simulink model "soc_estimation"  (R2024a)
settings: Solver=ode4  StartTime=0.0  StopTime=25000  FixedStep=0.001  MinStep=1e-3  RelTol=1e-3
values from neighbouring files (symbols this model uses):
  C1 = 1.6e-6    (= 1.6e-06)    [model_parameters.m]
  g = 9.8    [model_parameters.m]
  m = 860    [model_parameters.m]
  r = 0.33    [model_parameters.m]
  rho = 1.2    [model_parameters.m]
  S = 2.75    [model_parameters.m]
undefined symbols (not defined in the file or in its folder): C0, Cx
libraries: drivecyclelib x1
settings Model: Creator=marco  LastModifiedBy=QUDUS
settings SolverCC: AlgebraicLoopSolver=TrustRegion
settings DataIOCC: ReturnWorkspaceOutputs=off
settings DebuggingCC: UnconnectedInputMsg=warning  UnconnectedOutputMsg=warning  UnconnectedLineMsg=warning  UnderSpecifiedDimensionMsg=warning  ArithmeticOperatorsInVariantConditions=warning
settings ModelReferenceCC: EnableRefExpFcnMdlSchedulingChecks=on
settings SFSimCC: CustomCodeUndefinedFunction=UseInterfaceOnly
settings RTWCC: GPUComputeCapability=3.5

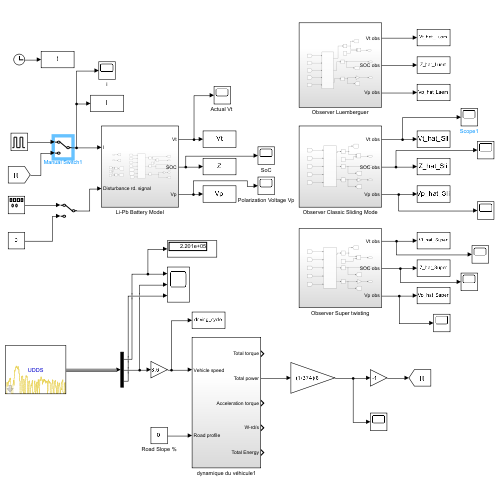
[thumbnail: Simulink's stored preview of the top-level diagram]
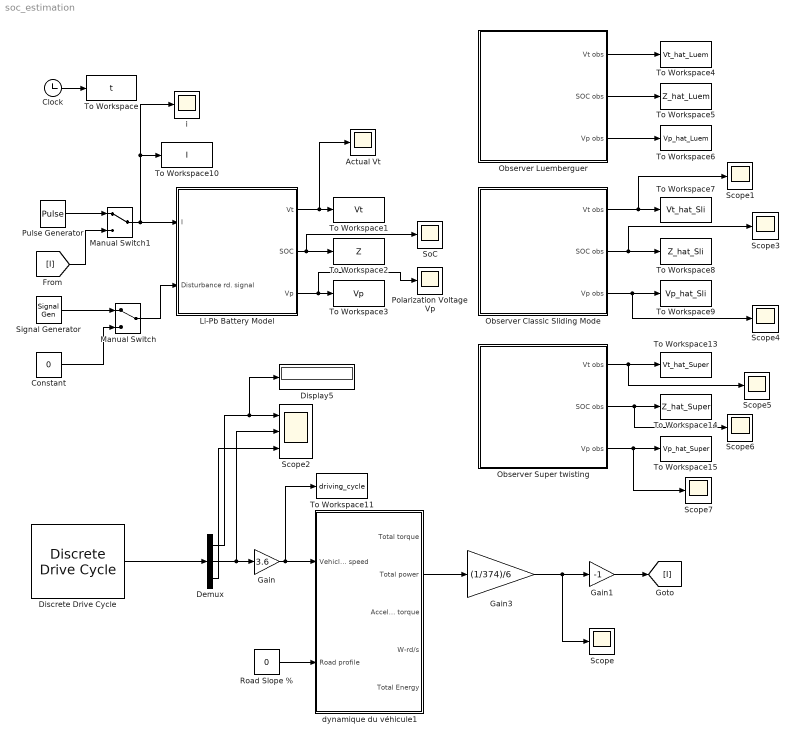
== system soc_estimation ==
  "Actual Vt " : Scope
  Clock : Clock
  Constant : Constant  Value=0
  Demux : Demux  Outputs=3
  Discrete Drive Cycle : drivecyclelib/Discrete Drive Cycle  CycleName=UDDS  CycleRepeatsForever=on  SampleTime=0.001
      settings: SourceProductName=Drive Cycles Blockset
  Display5 : Display
  Gain : Gain  Gain=3.6
  Gain1 : Gain  Gain=-1
  Gain3 : Gain  Gain=(1/374)/6
  Li-Pb Battery Model : Subsystem
  Manual Switch : ManualSwitch
  Manual Switch1 : ManualSwitch
  Observer Classic Sliding Mode : Subsystem
  Observer Luemberguer : Subsystem
  Observer Super twisting : Subsystem
  Polarization Voltage Vp : Scope
  Pulse Generator : DiscretePulseGenerator  PulseType=Time based  Amplitude=-5  Period=960  PulseWidth=(360*100)/960
  Road Slope % : Constant  Value=0
  Scope{,1,3..7} (7 alike) : Scope
  Scope2 : Scope  NumInputPorts=3
  Signal Generator : SignalGenerator  WaveForm=random  Amplitude=0.01  Frequency=1000
  SoC : Scope
  To Workspace : ToWorkspace  VariableName=t  SampleTime=-1
  To Workspace1 : ToWorkspace  VariableName=Vt  SampleTime=-1
  To Workspace10 : ToWorkspace  VariableName=I  SampleTime=-1
  To Workspace11 : ToWorkspace  VariableName=driving_cycle  SampleTime=-1
  To Workspace13 : ToWorkspace  VariableName=Vt_hat_Super  SampleTime=-1
  To Workspace14 : ToWorkspace  VariableName=Z_hat_Super  SampleTime=-1
  To Workspace15 : ToWorkspace  VariableName=Vp_hat_Super  SampleTime=-1
  To Workspace2 : ToWorkspace  VariableName=Z  SampleTime=-1
  To Workspace3 : ToWorkspace  VariableName=Vp  SampleTime=-1
  To Workspace4 : ToWorkspace  VariableName=Vt_hat_Luem  SampleTime=-1
  To Workspace5 : ToWorkspace  VariableName=Z_hat_Luem  SampleTime=-1
  To Workspace6 : ToWorkspace  VariableName=Vp_hat_Luem  SampleTime=-1
  To Workspace7 : ToWorkspace  VariableName=Vt_hat_Sli  SampleTime=-1
  To Workspace8 : ToWorkspace  VariableName=Z_hat_Sli  SampleTime=-1
  To Workspace9 : ToWorkspace  VariableName=Vp_hat_Sli  SampleTime=-1
  dynamique du véhicule1 : Subsystem
  i : Scope
  wires:
  Constant/1 -> Manual Switch/2
  Manual Switch/1 -> Li-Pb Battery Model/2(Disturbance rd. signal)
  Clock/1 -> To Workspace/1
  Li-Pb Battery Model/1(Vt) -> "Actual Vt "/1, To Workspace1/1
  Li-Pb Battery Model/3(Vp) -> Polarization Voltage Vp/1, To Workspace3/1
  Observer Luemberguer/1(Vt obs) -> To Workspace4/1
  Observer Luemberguer/2(SOC obs) -> To Workspace5/1
  Observer Luemberguer/3(Vp obs) -> To Workspace6/1
  Observer Classic Sliding Mode/2(SOC obs) -> Scope3/1, To Workspace8/1
  Observer Classic Sliding Mode/1(Vt obs) -> Scope1/1, To Workspace7/1
  Observer Classic Sliding Mode/3(Vp obs) -> Scope4/1, To Workspace9/1
  Observer Super twisting/3(Vp obs) -> Scope7/1, To Workspace15/1
  Observer Super twisting/2(SOC obs) -> Scope6/1, To Workspace14/1
  Observer Super twisting/1(Vt obs) -> Scope5/1, To Workspace13/1
  Signal Generator/1 -> Manual Switch/1
  Li-Pb Battery Model/2(SOC) -> SoC/1, To Workspace2/1
  Demux/3 -> Scope2/3
  Gain/1 -> To Workspace11/1, dynamique du véhicule1/1(Vehicle speed)
  Road Slope %/1 -> dynamique du véhicule1/2(Road profile)
  Discrete Drive Cycle/1 -> Demux/1
  Demux/2 -> Scope2/2, Gain/1
  Gain3/1 -> Gain1/1, Scope/1
  Demux/1 -> Display5/1, Scope2/1
  dynamique du véhicule1/2(Total power) -> Gain3/1
  Gain1/1 -> [I]
  Manual Switch1/1 -> i/1, To Workspace10/1, Li-Pb Battery Model/1(I)
  [I] -> Manual Switch1/2
  Pulse Generator/1 -> Manual Switch1/1

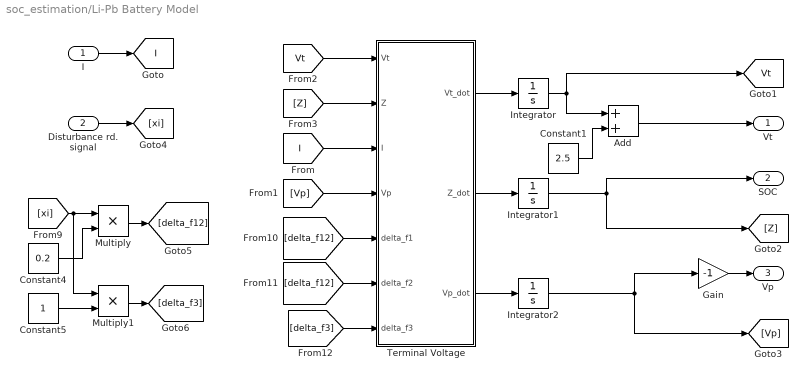
== system soc_estimation/Li-Pb Battery Model ==
  I : Inport
  Disturbance rd. signal : Inport  Port=2
  Add : Sum
  Constant1 : Constant  Value=2.5
  Constant4 : Constant  Value=0.2
  Constant5 : Constant
  Gain : Gain  Gain=-1
  Integrator : Integrator  InitialCondition=1.5
  Integrator1 : Integrator  InitialCondition=1
  Integrator2 : Integrator
  Multiply : Product
  Multiply1 : Product
  Terminal Voltage : MATLAB Function  TreatAsAtomicUnit=on
  Vt : Outport  VectorParamsAs1DForOutWhenUnconnected=off
  SOC : Outport  Port=2  VectorParamsAs1DForOutWhenUnconnected=off
  Vp : Outport  Port=3  VectorParamsAs1DForOutWhenUnconnected=off
  tag scope: I=global, Vt=global
  wires:
  I/1 -> [I]
  Disturbance rd. signal/1 -> [xi]
  [xi] -> Multiply1/1, Multiply/1
  Constant4/1 -> Multiply/2
  Constant5/1 -> Multiply1/2
  Multiply/1 -> [delta_f12]
  Multiply1/1 -> [delta_f3]
  [Vp] -> Terminal Voltage/4(Vp)
  [Vt] -> Terminal Voltage/1(Vt)
  Terminal Voltage/1(Vt_dot) -> Integrator/1
  [delta_f12] -> Terminal Voltage/6(delta_f2)
  [delta_f12] -> Terminal Voltage/5(delta_f1)
  Constant1/1 -> Add/2
  Add/1 -> Vt/1
  Integrator1/1 -> [Z], SOC/1
  Integrator2/1 -> [Vp], Gain/1
  Terminal Voltage/2(Z_dot) -> Integrator1/1
  [delta_f3] -> Terminal Voltage/7(delta_f3)
  Integrator/1 -> [Vt], Add/1
  Terminal Voltage/3(Vp_dot) -> Integrator2/1
  [Z] -> Terminal Voltage/2(Z)
  [I] -> Terminal Voltage/3(I)
  Gain/1 -> Vp/1

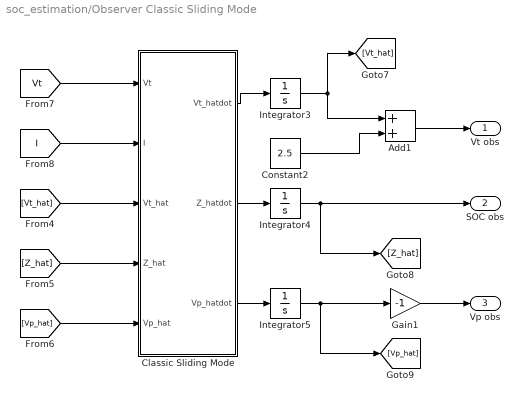
== system soc_estimation/Observer Classic Sliding Mode ==
  Add1 : Sum
  Classic Sliding Mode : MATLAB Function  TreatAsAtomicUnit=on
  Constant2 : Constant  Value=2.5
  Gain1 : Gain  Gain=-1
  Integrator3 : Integrator  InitialCondition=3
  Integrator4 : Integrator  InitialCondition=2
  Integrator5 : Integrator  InitialCondition=1
  Vt obs : Outport  VectorParamsAs1DForOutWhenUnconnected=off
  SOC obs : Outport  Port=2  VectorParamsAs1DForOutWhenUnconnected=off
  Vp obs : Outport  Port=3  VectorParamsAs1DForOutWhenUnconnected=off
  wires:
  Gain1/1 -> Vp obs/1
  [Z_hat] -> Classic Sliding Mode/4(Z_hat)
  Classic Sliding Mode/2(Z_hatdot) -> Integrator4/1
  Classic Sliding Mode/1(Vt_hatdot) -> Integrator3/1
  Integrator4/1 -> SOC obs/1, [Z_hat]
  Add1/1 -> Vt obs/1
  Integrator3/1 -> Add1/1, [Vt_hat]
  [Vt_hat] -> Classic Sliding Mode/3(Vt_hat)
  Constant2/1 -> Add1/2
  Classic Sliding Mode/3(Vp_hatdot) -> Integrator5/1
  [I] -> Classic Sliding Mode/2(I)
  Integrator5/1 -> Gain1/1, [Vp_hat]
  [Vp_hat] -> Classic Sliding Mode/5(Vp_hat)
  [Vt] -> Classic Sliding Mode/1(Vt)

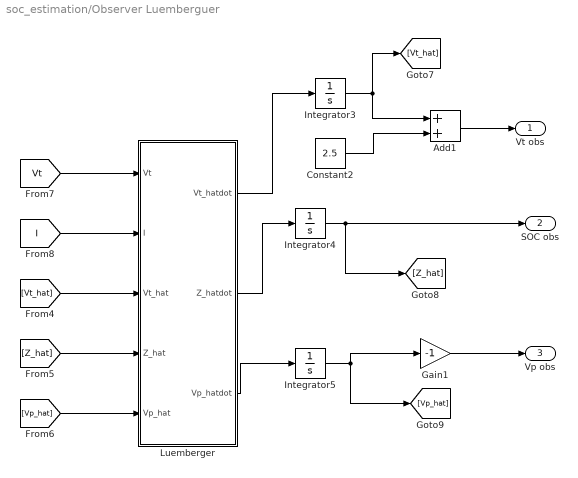
== system soc_estimation/Observer Luemberguer ==
  Add1 : Sum
  Constant2 : Constant  Value=2.5
  Gain1 : Gain  Gain=-1
  Integrator3 : Integrator  InitialCondition=3
  Integrator4 : Integrator  InitialCondition=2
  Integrator5 : Integrator  InitialCondition=1
  Luemberger : MATLAB Function  TreatAsAtomicUnit=on
  Vt obs : Outport  VectorParamsAs1DForOutWhenUnconnected=off
  SOC obs : Outport  Port=2  VectorParamsAs1DForOutWhenUnconnected=off
  Vp obs : Outport  Port=3  VectorParamsAs1DForOutWhenUnconnected=off
  wires:
  Gain1/1 -> Vp obs/1
  [Z_hat] -> Luemberger/4(Z_hat)
  Luemberger/2(Z_hatdot) -> Integrator4/1
  Luemberger/1(Vt_hatdot) -> Integrator3/1
  Integrator4/1 -> SOC obs/1, [Z_hat]
  Add1/1 -> Vt obs/1
  Integrator3/1 -> Add1/1, [Vt_hat]
  [Vt_hat] -> Luemberger/3(Vt_hat)
  Constant2/1 -> Add1/2
  Luemberger/3(Vp_hatdot) -> Integrator5/1
  [I] -> Luemberger/2(I)
  Integrator5/1 -> Gain1/1, [Vp_hat]
  [Vp_hat] -> Luemberger/5(Vp_hat)
  [Vt] -> Luemberger/1(Vt)

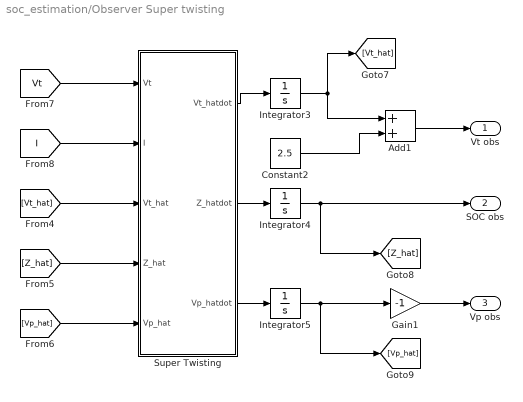
== system soc_estimation/Observer Super twisting ==
  Add1 : Sum
  Constant2 : Constant  Value=2.5
  Gain1 : Gain  Gain=-1
  Integrator3 : Integrator  InitialCondition=3
  Integrator4 : Integrator  InitialCondition=2
  Integrator5 : Integrator  InitialCondition=1
  Super Twisting : MATLAB Function  TreatAsAtomicUnit=on
  Vt obs : Outport  VectorParamsAs1DForOutWhenUnconnected=off
  SOC obs : Outport  Port=2  VectorParamsAs1DForOutWhenUnconnected=off
  Vp obs : Outport  Port=3  VectorParamsAs1DForOutWhenUnconnected=off
  wires:
  Gain1/1 -> Vp obs/1
  [Z_hat] -> Super Twisting/4(Z_hat)
  Super Twisting/2(Z_hatdot) -> Integrator4/1
  Super Twisting/1(Vt_hatdot) -> Integrator3/1
  Integrator4/1 -> SOC obs/1, [Z_hat]
  Add1/1 -> Vt obs/1
  Integrator3/1 -> Add1/1, [Vt_hat]
  [Vt_hat] -> Super Twisting/3(Vt_hat)
  Constant2/1 -> Add1/2
  Super Twisting/3(Vp_hatdot) -> Integrator5/1
  [I] -> Super Twisting/2(I)
  Integrator5/1 -> Gain1/1, [Vp_hat]
  [Vp_hat] -> Super Twisting/5(Vp_hat)
  [Vt] -> Super Twisting/1(Vt)

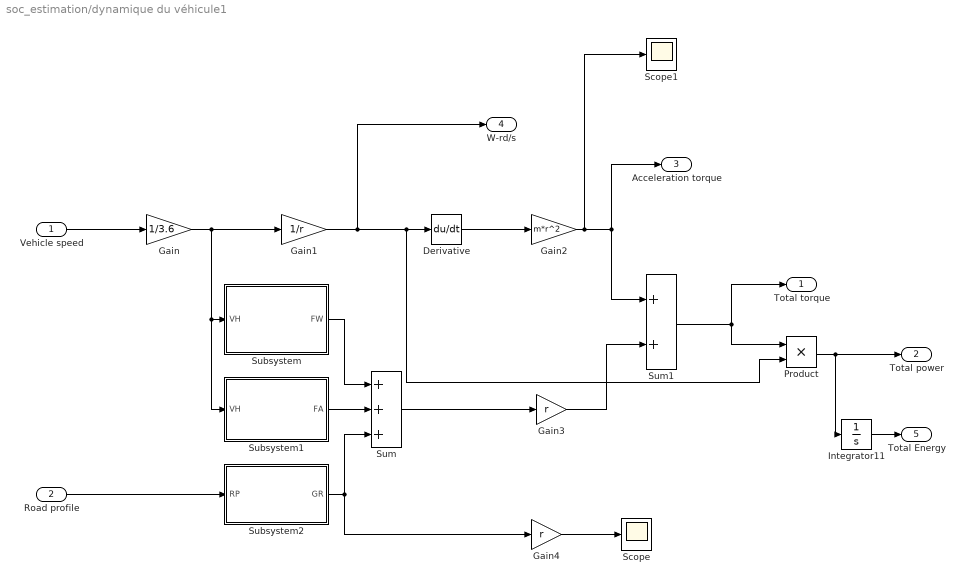
== system soc_estimation/dynamique du véhicule1 ==
  Vehicle speed : Inport
  Road profile : Inport  Port=2
  Derivative : Derivative
  Gain : Gain  Gain=1/3.6
  Gain1 : Gain  Gain=1/r
  Gain2 : Gain  Gain=m*r^2
  Gain3 : Gain  Gain=r
  Gain4 : Gain  Gain=r
  Integrator11 : Integrator
  Product : Product
  Scope : Scope
  Scope1 : Scope
  Subsystem : Subsystem
  Subsystem1 : Subsystem
  Subsystem2 : Subsystem
  Sum : Sum  Inputs=+++
  Sum1 : Sum
  Total torque : Outport  VectorParamsAs1DForOutWhenUnconnected=off
  Total power : Outport  Port=2  VectorParamsAs1DForOutWhenUnconnected=off
  Acceleration torque : Outport  Port=3  VectorParamsAs1DForOutWhenUnconnected=off
  W-rd/s : Outport  Port=4  VectorParamsAs1DForOutWhenUnconnected=off
  Total Energy : Outport  Port=5  VectorParamsAs1DForOutWhenUnconnected=off
  wires:
  Integrator11/1 -> Total Energy/1
  Vehicle speed/1 -> Gain/1
  Gain/1 -> Subsystem1/1(VH), Subsystem/1(VH), Gain1/1
  Road profile/1 -> Subsystem2/1(RP)
  Gain1/1 -> W-rd/s/1, Derivative/1, Product/2
  Derivative/1 -> Gain2/1
  Subsystem/1(FW) -> Sum/1
  Subsystem1/1(FA) -> Sum/2
  Subsystem2/1(GR) -> Gain4/1, Sum/3
  Sum/1 -> Gain3/1
  Gain4/1 -> Scope/1
  Gain2/1 -> Scope1/1, Acceleration torque/1, Sum1/1
  Gain3/1 -> Sum1/2
  Sum1/1 -> Total torque/1, Product/1
  Product/1 -> Integrator11/1, Total power/1

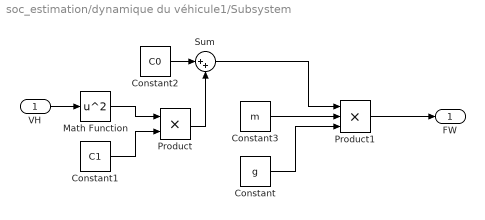
== system soc_estimation/dynamique du véhicule1/Subsystem ==
  VH : Inport
  Constant : Constant  Value=g
  Constant1 : Constant  Value=C1
  Constant2 : Constant  Value=C0
  Constant3 : Constant  Value=m
  Math Function : Math  Operator=square  SignedPower=on
  Product : Product
  Product1 : Product  Inputs=3
  Sum : Sum  Inputs=|++
  FW : Outport
  wires:
  Math Function/1 -> Product/1
  Constant3/1 -> Product1/2
  VH/1 -> Math Function/1
  Constant2/1 -> Sum/1
  Product/1 -> Sum/2
  Constant1/1 -> Product/2
  Product1/1 -> FW/1
  Constant/1 -> Product1/3
  Sum/1 -> Product1/1

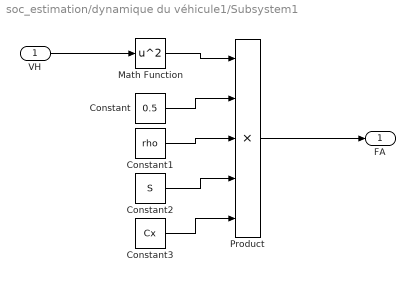
== system soc_estimation/dynamique du véhicule1/Subsystem1 ==
  VH : Inport
  Constant : Constant  Value=0.5
  Constant1 : Constant  Value=rho
  Constant2 : Constant  Value=S
  Constant3 : Constant  Value=Cx
  Math Function : Math  Operator=square  SignedPower=on
  Product : Product  Inputs=5
  FA : Outport
  wires:
  Constant1/1 -> Product/3
  Constant/1 -> Product/2
  Product/1 -> FA/1
  Math Function/1 -> Product/1
  Constant2/1 -> Product/4
  Constant3/1 -> Product/5
  VH/1 -> Math Function/1

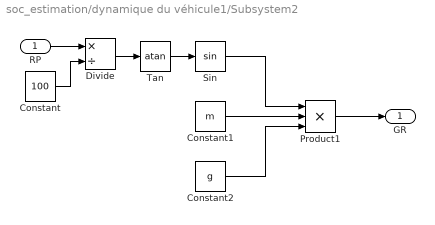
== system soc_estimation/dynamique du véhicule1/Subsystem2 ==
  RP : Inport
  Constant : Constant  Value=100
  Constant1 : Constant  Value=m
  Constant2 : Constant  Value=g
  Divide : Product  Inputs=*/
  Product1 : Product  Inputs=3
  Sin : Trigonometry
  Tan : Trigonometry  Operator=atan
  GR : Outport
  wires:
  Sin/1 -> Product1/1
  RP/1 -> Divide/1
  Constant/1 -> Divide/2
  Divide/1 -> Tan/1
  Constant1/1 -> Product1/2
  Product1/1 -> GR/1
  Constant2/1 -> Product1/3
  Tan/1 -> Sin/1

== matlab function soc_estimation/Li-Pb Battery Model/Terminal Voltage ==
  data: Vt input; Vt_dot output; Z input; I input; Vp input; delta_f1 input; delta_f2 input; delta_f3 input; Z_dot output; Vp_dot output
function [Vt_dot,Z_dot,Vp_dot] = fcn(Vt,Z,I,Vp,delta_f1,delta_f2,delta_f3)
%---------------------- RC battery model parameters ----------------------
K = 1.7;                       % Linear relationship
%Cp = 200;                      % Capacitance [F]
%Rp = 0.003;                    % Diffusion resistance [ohm]
%Rt = 0.001;                    % Ohmic resistance [ohm]
%Cn = 5;                      % Nominal capacity [Ah]

%%%%%%%%%%%%%%%%%%%%%% Linear model parameters %%%%%%%%%%%%%%%%%%%%%%
%a1 = 1/(Rp*Cp); 
%a2 = 1/(Rt*Cn); 
%b1 = (1/Cn) + (1/Cp) + (Rt/(Rp*Cp));
%b2 = 1/Cp;

a1 = 1.667; 
a2 = 0.0589;
b1 = 0.00672;
b2 = 0.005;
a11= 2.8339;
a22= 0.1001;

Vt_dot = -a1*Vt + a1*K*Z + b1*I + delta_f1;
Z_dot = a2*Vt - a2*K*Z - a2*Vp + delta_f2;
Vp_dot = -a1*Vp + b2*I + delta_f3;

== matlab function soc_estimation/Observer Luemberguer/Luemberger ==
  data: Vt input; I input; Vt_hatdot output; Vt_hat input; Z_hat input; Vp_hat input; Z_hatdot output; Vp_hatdot output
function [Vt_hatdot,Z_hatdot,Vp_hatdot] = fcn(Vt,I,Vt_hat,Z_hat,Vp_hat)

% We have to build the observer in the form:
% X_hatdot = A*X_hat + B*u + H*(y-y_hat) + rho*gamma*sign(y-y_hat)

K = 1.7; 

a1 = 1.667; 
a2 = 0.0589; 
b1 = 0.00672;
b2 = 0.005;
a11= 2.8339;
a22= 0.1001;


err = (Vt - Vt_hat);

%H = [h1; h2; h3]; % gain matrix
h1 = 1.3629;
h2 = 0.9530;
h3 = -0.0046;

rho = 0.2;
gamma1 = 0.2;
gamma2 = 0.2;
gamma3 = 1;

% Vt_hatdot = -a1*Vt_hat + a1*K*Z_hat + b1*I + h1*(abs(err)^(2/3))*sign(err); %+ rho*gamma1*sign(err);
% Z_hatdot = a2*Vt_hat - a2*K*Z_hat - a2*Vp_hat + h2*(abs(err)^(1/3))*sign(err);%+ rho*gamma2*sign(err);
% Vp_hatdot = -a1*Vp_hat + b2*I + h3*sign(err); %+ rho*gamma3*sign(err); 

%Vt_hatdot = -a1*Vt_hat + a1*K*Z_hat + b1*I + h1*err + rho*gamma1*sign(err);
%Z_hatdot = a2*Vt_hat - a2*K*Z_hat - a2*Vp_hat + h2*err + rho*gamma2*sign(err);
%Vp_hatdot = -a1*Vp_hat + b2*I + h3*err + rho*gamma3*sign(err);

Vt_hatdot = -a1*Vt_hat + a1*K*Z_hat + b1*I + h1*err;
Z_hatdot = a2*Vt_hat - a2*K*Z_hat - a2*Vp_hat + h2*err;
Vp_hatdot = -a1*Vp_hat + b2*I + h3*err;

== matlab function soc_estimation/Observer Classic Sliding Mode/Classic Sliding Mode ==
  data: Vt input; I input; Vt_hatdot output; Vt_hat input; Z_hat input; Vp_hat input; Z_hatdot output; Vp_hatdot output
function [Vt_hatdot,Z_hatdot,Vp_hatdot] = fcn(Vt,I,Vt_hat,Z_hat,Vp_hat)

% We have to build the observer in the form:
% X_hatdot = A*X_hat + B*u + H*(y-y_hat) + rho*gamma*sign(y-y_hat)

K = 1.7; 

a1 = 1.667; 
a2 = 0.0589; 
b1 = 0.00672;
b2 = 0.005;
a11= 2.8339;
a22= 0.1001;


err=(Vt - Vt_hat);

%H = [h1; h2; h3]; % gain matrix
h1 = 1.3629;
h2 = 0.9530;
h3 = -0.0046;

rho = 0.2;
gamma1 = 0.2;
gamma2 = 0.2;
gamma3 = 1;

% Vt_hatdot = -a1*Vt_hat + a1*K*Z_hat + b1*I + h1*(abs(err)^(2/3))*sign(err); %+ rho*gamma1*sign(err);
% Z_hatdot = a2*Vt_hat - a2*K*Z_hat - a2*Vp_hat + h2*(abs(err)^(1/3))*sign(err);%+ rho*gamma2*sign(err);
% Vp_hatdot = -a1*Vp_hat + b2*I + h3*sign(err); %+ rho*gamma3*sign(err); 

Vt_hatdot = -a1*Vt_hat + a1*K*Z_hat + b1*I + h1*sign(err); %+ rho*gamma1*sign(err);
Z_hatdot = a2*Vt_hat - a2*K*Z_hat - a2*Vp_hat + h2*sign(err); %+ rho*gamma2*sign(err);
Vp_hatdot = -a1*Vp_hat + b2*I + h3*sign(err); %+ rho*gamma3*sign(err); 

%Vt_hatdot = -a1*Vt_hat + a1*K*Z_hat + b1*I + h1*err + rho*gamma1*sign(err);
%Z_hatdot = a2*Vt_hat - a2*K*Z_hat - a2*Vp_hat + h2*err + rho*gamma2*sign(err);
%Vp_hatdot = -a1*Vp_hat + b2*I + h3*err + rho*gamma3*sign(err);

== matlab function soc_estimation/Observer Super twisting/Super Twisting ==
  data: Vt input; I input; Vt_hatdot output; Vt_hat input; Z_hat input; Vp_hat input; Z_hatdot output; Vp_hatdot output
function [Vt_hatdot,Z_hatdot,Vp_hatdot] = fcn(Vt,I,Vt_hat,Z_hat,Vp_hat)

% We have to build the observer in the form:
% X_hatdot = A*X_hat + B*u + H*(y-y_hat) + rho*gamma*sign(y-y_hat)

K = 1.7; 

a1 = 1.667; 
a2 = 0.0589; 
b1 = 0.00672;
b2 = 0.005;
a11= 2.8339;
a22= 0.1001;


err=(Vt - Vt_hat);

%H = [h1; h2; h3]; % gain matrix
h1 = 1.3629;
h2 = 0.9530;
h3 = -0.0046;

rho = 0.2;
gamma1 = 0.2;
gamma2 = 0.2;
gamma3 = 1;

Vt_hatdot = -a1*Vt_hat + a1*K*Z_hat + b1*I + h1*(abs(err)^(2/3))*sign(err); %+ rho*gamma1*sign(err);
Z_hatdot = a2*Vt_hat - a2*K*Z_hat - a2*Vp_hat + h2*(abs(err)^(1/3))*sign(err);%+ rho*gamma2*sign(err);
Vp_hatdot = -a1*Vp_hat + b2*I + h3*sign(err); %+ rho*gamma3*sign(err); 

%Vt_hatdot = -a1*Vt_hat + a1*K*Z_hat + b1*I + h1*err + rho*gamma1*(abs(err)^(2/3))*sign(err);
%Z_hatdot = a2*Vt_hat - a2*K*Z_hat - a2*Vp_hat + h2*err + rho*gamma2*(abs(err)^(1/3))*sign(err);
%Vp_hatdot = -a1*Vp_hat + b2*I + h3*err + rho*gamma3*sign(err);
